simulink model "SensorSupply_harness"  (Simulink 7.7)
settings: Solver=FixedStepDiscrete  SolverMode=SingleTasking  StartTime=0.0  StopTime=100  FixedStep=.1  RelTol=1e-3
PostLoadFcn:
  | PostLoadFcn2;
InitFcn:
  | if signalbuilder('SensorSupply_harness/Signal_Builder','activegroup') == 2
  |   CD_SENSOR_SUPPLY1_FUNCTION.DataType = 'uint8';
  |   CD_SENSOR_SUPPLY1_FUNCTION.Value = 255;
  | else
  |   CD_SENSOR_SUPPLY1_FUNCTION.DataType = 'uint8';
  |   CD_SENSOR_SUPPLY1_FUNCTION.Value = 0;
  | end
undefined symbols (not defined in the file): CD_SENSOR_SUPPLY1_DEBOUNCE_NORMAL, CD_SENSOR_SUPPLY1_DEBOUNCE_OORH, CD_SENSOR_SUPPLY1_DEBOUNCE_OORL, CD_SENSOR_SUPPLY1_OORH, CD_SENSOR_SUPPLY1_OORL, NON_FUNCTIONAL, NORMAL, OORH, OORL, sigbuilder_block, srate100
settings Model: Creator=smindema  LastModifiedBy=aliebel  RecordCoverage=on  CovMetricSettings=dcmw  CovCumulativeReport=on
settings MATStruct: SampleTime=0.01  Offset=0  Priority=[1.0]
settings DataIOCC: LimitDataPoints=off  SaveOutput=off  SaveTime=off
settings OptimizationCC: BlockReduction=off  InlineParams=on  ExpressionFolding=off  StateBitsets=on  DataBitsets=on  UseTempVars=on  InitFltsAndDblsToZero=on  NoFixptDivByZeroProtection=on  EfficientFloat2IntCast=on  OptimizeModelRefInitCode=on
settings DebuggingCC: SaveWithParameterizedLinksMsg=none  MultiTaskDSMMsg=warning  MultiTaskCondExecSysMsg=none  IntegerOverflowMsg=none  ModelReferenceCSMismatchMessage=warning
settings HardwareCC: ProdBitPerInt=16  ProdBitPerPointer=16  ProdIntDivRoundTo=Floor  ProdEndianess=BigEndian  ProdWordSize=16  ProdHWDeviceType=Motorola HC12
settings ModelReferenceCC: ModelReferenceNumInstancesAllowed=Single
settings RTWCC: SystemTargetFile=ert.tlc  GenCodeOnly=on  TemplateMakefile=ert_default_tmf  Description=Real-Time Workshop Embedded Coder (no auto configuration)  GenerateReport=on  RetainRTWFile=on  ProcessScript=ert_make_rtw_hook  IncludeHyperlinkInReport=on  LaunchReport=on  IncludeERTFirstTime=on
settings RTWCC: CustomHeaderCode=|
  | #include "cpp_req_defines.h"
  | #include "hw_fin.h"
  | #include "cdata.h"
settings CodeAppCC: IgnoreCustomStorageClasses=off  DefineNamingRule=UpperCase
settings ERTTargetCC: TargetFcnLib=ansi_tfl_tmw.mat  FunctionExecutionProfile=off  MultiwordLength=2048  GenerateSampleERTMain=on  IncludeMdlTerminateFcn=off  SupportAbsoluteTime=off  SupportNonFinite=off  SupportComplex=off  PurelyIntegerCode=on  ERTCustomFileTemplate=gen_rtw_req_defines_h.tlc  GlobalDataDefinition=InSeparateSourceFile  GlobalDataReference=InSeparateHeaderFile  ConvertIfToSwitch=off

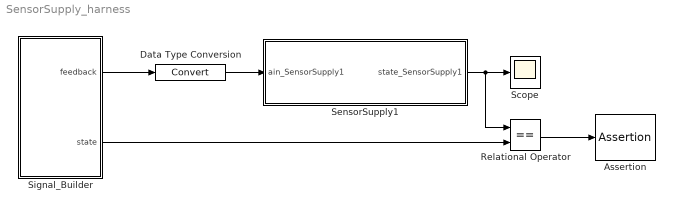
== system SensorSupply_harness ==
  Assertion : Assertion  Enabled=on
  Data Type Conversion : DataTypeConversion
  Relational Operator : RelationalOperator  Operator===  OutDataTypeStr=boolean
  Scope : Scope
      settings: YMin=8  YMax=22
  SensorSupply1 : Subsystem  TreatAsAtomicUnit=on  SystemSampleTime=srate100  RTWFileName=mod_Inputs
      settings: RTWSystemCode=Function  RTWFcnNameOpts=Use subsystem name  RTWFileNameOpts=User specified
  Signal_Builder : Subsystem  Tag=STV Subsys  LoadFcn=sigbuilder_block('load');  StartFcn=sigbuilder_block('start');  StopFcn=sigbuilder_block('stop');  ClipboardFcn=sigbuilder_block('clipboard');  mask(Sigbuilder block){}
      mask help: Sigbuilder GUI
      mask init:
      | if ~strcmp(get_param(bdroot(gcbh),'SimulationStatus'),'stopped') tuvar = sigbuilder_block('maskInit'); end
      settings: CopyFcn=sigbuilder_block('copy');  DeleteFcn=sigbuilder_block('delete');  ModelCloseFcn=sigbuilder_block('modelClose');  PreSaveFcn=sigbuilder_block('preSave');  NameChangeFcn=sigbuilder_block('namechange');  OpenFcn=sigbuilder_block('open',[411.75 204.75 732.75 548.25 ]);  CloseFcn=sigbuilder_block('close');
      mask Display: plot(0,0,100,100,[10,10,40,40,10],[80,20,20,80,80],[40,10],[50,50], [40,27,10],[65,72,56],[40,25,25,10],[28,28,43,43]);
  wires:
  Data Type Conversion/1 -> SensorSupply1/1(ain_SensorSupply1)
  SensorSupply1/1(state_SensorSupply1) -> Scope/1, Relational Operator/1
  Signal_Builder/1(feedback) -> Data Type Conversion/1
  Relational Operator/1 -> Assertion/1
  Signal_Builder/2(state) -> Relational Operator/2

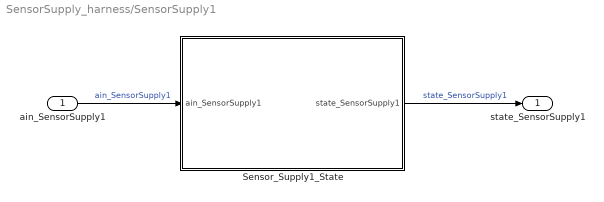
== system SensorSupply_harness/SensorSupply1 ==
  ain_SensorSupply1 : Inport  OutDataTypeStr=uint16
  Sensor_Supply1_State : Stateflow chart  TreatAsAtomicUnit=on
  state_SensorSupply1 : Outport  OutDataTypeStr=uint8
  wires:
  Sensor_Supply1_State/1(state_SensorSupply1) -> state_SensorSupply1/1  "state_SensorSupply1"
  ain_SensorSupply1/1 -> Sensor_Supply1_State/1(ain_SensorSupply1)  "ain_SensorSupply1"

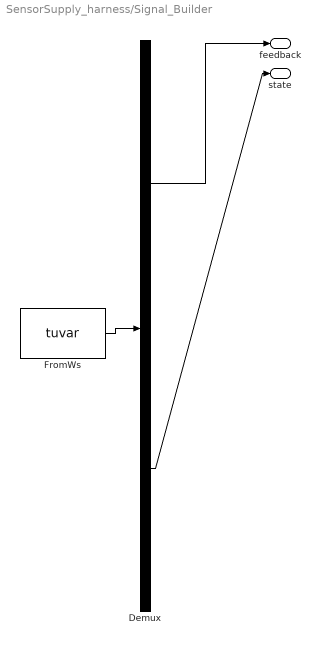
== system SensorSupply_harness/Signal_Builder ==
  Demux : Demux  Tag=STV Demux  Outputs=2
  FromWs : FromWorkspace  Tag=STV FromWs  VariableName=tuvar  SampleTime=0  SigBuilderData=DataTag0  VnvData=DataTag1
      SigBuilderData=|
      | common.afterFinalStr = 'Extrapolate'
      | common.sampleTime = 0
      | dataSet(1).timeRange = [0 100]
      | dataSet(1).name = 'Group 1'
      | dataSet(2).timeRange = [0 100]
      | dataSet(2).name = 'NONFUNCTIONAL'
      | sbobj.Groups(1).Name = 'Group 1'
      | sbobj.Groups(1).Signals(1).Name = 'feedback'
      | sbobj.Groups(1).Signals(1).XData = [0 20 20 20.2 20.2 27 27 34 34 34.3 34.3 40 40 44 44 44.01 44.01 60 60 60.02 60.02 62.6 62.6 70 70 70.2 70.2 75 75 100]
      | sbobj.Groups(1).Signals(1).YData = [850 850 946 946 850 850 947 947 850 850 946 946 850 850 946 946 850 850 760 760 850 850 760 760 860 860 760 760 850 850]
      | sbobj.Groups(1).Signals(2).Name = 'state'
      | sbobj.Groups(1).Signals(2).XData = [0 32.1 32.1 49.2 49.2 67.7 67.7 80.1 80.1 100]
      | sbobj.Groups(1).Signals(2).YData = [8 8 21 21 8 8 22 22 8 8]
      | sbobj.Groups(2).Name = 'NONFUNCTIONAL'
      | sbobj.Groups(2).Signals(1).Name = 'feedback'
      | sbobj.Groups(2).Signals(1).XData = [0 20 20 20.2 20.2 27 27 34 34 34.3 34.3 40 40 44 44 44.01 44.01 60 60 60.02 60.02 62.6 62.6 69.8 69.8 70 70 75 75 100]
      | sbobj.Groups(2).Signals(1).YData = [850 850 946 946 850 850 947 947 850 850 946 946 850 850 946 946 850 850 760 760 850 850 760 760 860 860 760 760 850 850]
      | sbobj.Groups(2).Signals(2).Name = 'state'
      | sbobj.Groups(2).Signals(2).XData = [0 32.4 100]
      | sbobj.Groups(2).Signals(2).YData = [8 8 8]
  feedback : Outport  Tag=STV Outport
  state : Outport  Tag=STV Outport  Port=2
  wires:
  Demux/1 -> feedback/1
  FromWs/1 -> Demux/1
  Demux/2 -> state/1

== stateflow chart SensorSupply1/Sensor_Supply1_State ==
  state NON_FUNCTIONAL
    en:state_SensorSupply1 = NORMAL;
  state NORMAL
    state Debounce
      en:debounceCount = 0;
      du:debounceCount++
    state NORMAL
      en:state_SensorSupply1 = NORMAL;
    NORMAL.Debounce -> NORMAL.NORMAL : [(debounceCount >= CD_SENSOR_SUPPLY1_DEBOUNCE_NORMAL)...
        | || (state_SensorSupply1 == NORMAL)]
    (default) -> NORMAL.Debounce
  state OORL
    state NORMAL
      en:state_SensorSupply1 = OORL;
    state Debounce
      en:debounceCount = 0;
      du:debounceCount++
    OORL.Debounce -> OORL.NORMAL : [(debounceCount >= CD_SENSOR_SUPPLY1_DEBOUNCE_OORL)...
        | || (state_SensorSupply1 == OORL)]
    (default) -> OORL.Debounce
  state OORH
    state Debounce
      en:debounceCount = 0;
      du:debounceCount++
    state OORH
      en:state_SensorSupply1 = OORH;
    OORH.Debounce -> OORH.OORH : [(debounceCount >= CD_SENSOR_SUPPLY1_DEBOUNCE_OORH)...
        | || (state_SensorSupply1 == OORH)]
    (default) -> OORH.Debounce
  NON_FUNCTIONAL -> NORMAL : [(CD_SENSOR_SUPPLY1_FUNCTION != NON_FUNCTIONAL)]
  OORL -> NORMAL : [(ain_SensorSupply1 > CD_SENSOR_SUPPLY1_OORL)]
  NORMAL -> OORL [order 1] : [(ain_SensorSupply1 <= CD_SENSOR_SUPPLY1_OORL)]
  OORH -> NORMAL : [(ain_SensorSupply1 < CD_SENSOR_SUPPLY1_OORH)]
  NORMAL -> OORH [order 2] : [(ain_SensorSupply1 >= CD_SENSOR_SUPPLY1_OORH)]
  (default) -> NON_FUNCTIONAL
  data: state_SensorSupply1 output uint8; ain_SensorSupply1 input uint16; CD_SENSOR_SUPPLY1_FUNCTION parameter uint8; CD_SENSOR_SUPPLY1_OORL parameter uint16; CD_SENSOR_SUPPLY1_OORH parameter uint16; CD_SENSOR_SUPPLY1_DEBOUNCE_NORMAL parameter uint16; CD_SENSOR_SUPPLY1_DEBOUNCE_OORH parameter uint16; CD_SENSOR_SUPPLY1_DEBOUNCE_OORL parameter uint16; debounceCount local uint16 =0; OORH parameter uint8 =21; OORL parameter uint8 =22; NON_FUNCTIONAL parameter uint8 =255; NORMAL parameter uint8 =8
